simulink model "ds1_inter"  (R2019a)
settings: Solver=ode14x  StartTime=beginTime  StopTime=0.166  FixedStep=1e-4  RelTol=1e-3  EnableMultiTasking=on
model workspace (MAT data in the model file):
  Ankle_L_D = 0.125126243033
  Ankle_L_S = 0.0328154604487
  Ankle_R_D = 0.245807097642
  Ankle_R_S = 0.0328154604487
  F_C = 0.0618
  F_H = 0.107
  F_I = 0.0103200285075
  F_L = 0.2471
  F_M = 1.2499
  F_W = 0.11
  GRF_HD = 941.037069119
  GRF_HS = 1691.11560066
  GRF_VD = 12300.8672242
  GRF_VS = 76710.3574634
  HAT_I = 5.06801
  HAT_L = 0.549
  HAT_M = 58.9182
  HAT_a = 0.2
  HAT_b = 0.13
  Hip_L_D = 0.0332143791481
  Hip_L_S = 0.0516603438036
  Hip_R_D = 0.145088103411
  Hip_R_S = 0.15911410017
  Knee_L_D = 0.0558982452805
  Knee_L_S = 0.00250387295429
  Knee_R_D = 0.0619293882143
  Knee_R_S = 0.0623339259595
  M : struct (value not decoded)
  Planar_joint_x_p_i = 0
  Planar_joint_x_v_i = 0
  Planar_joint_y_p_i = 0
  Planar_joint_y_v_i = 0
  Planar_joint_z_p_i = -10.3139246991
  Planar_joint_z_w_i = -47.4942945829
  S_I = 0.0584148214017
  S_L = 0.447
  S_M = 4.0083
  S_R1 = 0.06
  S_R2 = 0.08
  T_I = 0.243990929891
  T_L = 0.476
  T_M = 8.62
  T_R1 = 0.08
  T_R2 = 0.1
  beginTime = 0
  bodymass = 86.2
  lagStanceAnkle = [0 0 0 0 0 0]
  lagStanceKnee = [0 0 0 0 0 0]
  lagSwingAnkle = [0 0 0 0 0 0]
  lagSwingKnee = [0 0 0 0 0 0]
  p_stance_ankle_i = 14.9539905036
  p_stance_hip_i = -24.9413676415
  p_stance_knee_i = -2.50807459996
  p_swing_ankle_i = 4.11757124464
  p_swing_hip_i = 18.3000604838
  p_swing_knee_i = -3.41741510381
  polyfit_stance_ankle = [-863347.977095 222377.922877 -7468.35453889 -9.40558010807 -153.06789694]
  polyfit_stance_hip = [-279786636.688 114363391.625 -15725654.0525 856134.662579 -22930.0516399 481.110496147 63.2694363354]
  polyfit_stance_knee = [-122862314.114 52903969.6705 -7988612.27678 487806.049871 -8969.32141641 330.337585729 -54.0526736443]
  polyfit_swing_ankle = [49510154320.8 -30205907167.6 7312588550.85 -888915044.437 56385922.5861 -1769074.37171 25613.4020917 -113.306543933 -1.03720591697]
  polyfit_swing_hip = [538683495113 -366532634246 101719653645 -14750073882.9 1184454520.37 -50949861.1242 1019832.60417 -6310.84925925 -38.0907282261]
  polyfit_swing_knee = [352478408737 -233011269241 62650744932.5 -8775138187.04 678489689.503 -28060179.8998 545151.783137 -3282.03325692 -26.455631467]
  time = [0 0.00833333333333 0.0166666666667 0.025 0.0333333333333 0.0416666666667 0.05 0.0583333333333 0.0666666666667 0.075 0.0833333333333 0.0916666666667 ... (21 elements, 21x1)]
  w_stance_ankle_i = 4.51440934049
  w_stance_hip_i = 2.37738035886
  w_stance_knee_i = 12.74290384
  w_swing_ankle_i = -56.5478745686
  w_swing_hip_i = 68.5572835202
  w_swing_knee_i = 17.3722348151
values from neighbouring files (symbols this model uses):
  N = 3    [lagdmodel.m]
symbols that are objects in the model workspace (value not decoded): M
undefined symbols (not defined in the file or in its folder): X, Y, Z
libraries: nesl_utility x59, sm_lib x49, fl_lib x24, fl_ps_legacy_lib x14, simulink x4
(part 2 of 3)

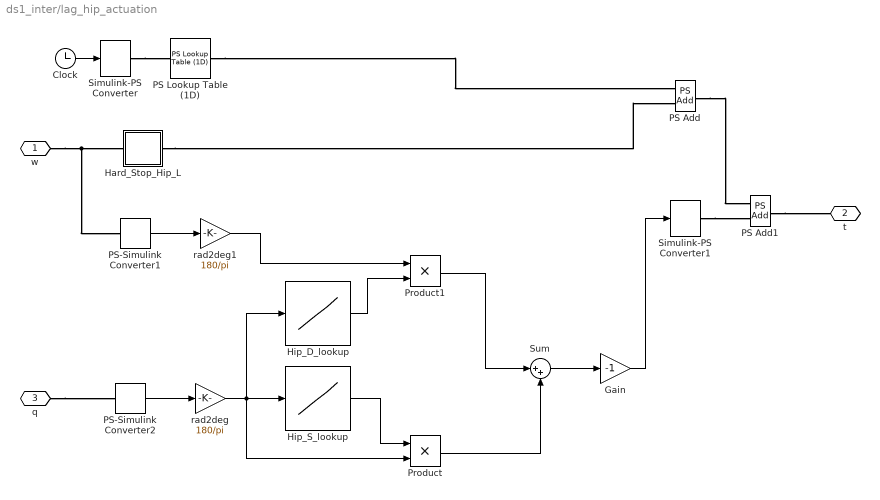
== system ds1_inter/lag_hip_actuation ==
  Clock : Clock
  Gain : Gain  Gain=-1
  Hard_Stop_Hip_L : Subsystem  mask{upper_bound=((125-p_stance_hip_i)*pi)/180, lower_bound=((-30-p_stance_hip_i)*pi)/180, contact_stiffness=1e8, contact_damping=5000, initial_angular_position=0}
      mask prompts: upper_bound "Upper Bound"; lower_bound "Lower Bound"; contact_stiffness "Contact Stiffness"; contact_damping "Contact Damping"; initial_angular_position "Initial Angular Position"
  Hip_D_lookup : Lookup_n-D  NumberOfTableDimensions=1  BreakpointsForDimension1=[-30:.01:125]  Table=[exp(linspace(log(1000),log(.01),1000)), zeros(1,13500),exp(linspace(log(.01),log(1000),1001))]  RndMeth=Simplest  InputSameDT=on
  Hip_S_lookup : Lookup_n-D  NumberOfTableDimensions=1  BreakpointsForDimension1=[-30:.01:125]  Table=[exp(linspace(log(10000),log(.01),1000)), zeros(1,13500),exp(linspace(log(.01),log(10000),1001))]  RndMeth=Simplest  InputSameDT=on
  PS Add : fl_ps_legacy_lib/Legacy Physical Signals/Functions/PS Add
      settings: SourceProductName=Simscape  SourceProductBaseCode=SS
  PS Add1 : fl_ps_legacy_lib/Legacy Physical Signals/Functions/PS Add
      settings: SourceProductName=Simscape  SourceProductBaseCode=SS
  PS Lookup Table (1D) : fl_ps_legacy_lib/Legacy Physical Signals/Lookup Tables/PS Lookup Table (1D)  x=linspace(0,.1667,21)'  f=(-M.stance_hip/1000)*bodymass  interp_method=2  extrap_method=1
      settings: SourceProductName=Simscape  SourceProductBaseCode=SS
  PS-Simulink Converter1 : nesl_utility/PS-Simulink Converter  PhysicalDomain=network_engine_domain  SubClassName=ps_output  LeftPortType=input  RightPortType=output  PseudoPeriodic=off  Frequencies=[]  Unit=1  AffineConversion=off
  PS-Simulink Converter2 : nesl_utility/PS-Simulink Converter  PhysicalDomain=network_engine_domain  SubClassName=ps_output  LeftPortType=input  RightPortType=output  PseudoPeriodic=off  Frequencies=[]  Unit=1  AffineConversion=off
  Product : Product  RndMeth=Zero
  Product1 : Product  RndMeth=Zero
  Simulink-PS Converter : nesl_utility/Simulink-PS Converter  PhysicalDomain=network_engine_domain  SubClassName=ps_input  LeftPortType=input  RightPortType=output  PseudoPeriodic=off  Frequencies=[]  NoiseDistribution=none  NoiseParameters=[]  Unit=1  AffineConversion=off  FilteringAndDerivatives=zero  SimscapeFilterOrder=1  InputFilterTimeConstant=.001  UdotUserProvided=[]
  Simulink-PS Converter1 : nesl_utility/Simulink-PS Converter  PhysicalDomain=network_engine_domain  SubClassName=ps_input  LeftPortType=input  RightPortType=output  PseudoPeriodic=off  Frequencies=[]  NoiseDistribution=none  NoiseParameters=[]  Unit=1  AffineConversion=off  FilteringAndDerivatives=zero  SimscapeFilterOrder=1  InputFilterTimeConstant=.001  UdotUserProvided=[]
  Sum : Sum  Inputs=|++
  rad2deg : Gain  Gain=180/pi
  "rad2deg1 " : Gain  Gain=180/pi
  w : PMIOPort  Side=Right
  t : PMIOPort  Port=2  Side=Left
  q : PMIOPort  Port=3  Side=Right
  wires:
  PS-Simulink Converter1/1 -> "rad2deg1 "/1
  PS-Simulink Converter2/1 -> rad2deg/1
  rad2deg/1 -> Hip_S_lookup/1, Hip_D_lookup/1, Product/2
  Hip_S_lookup/1 -> Product/1
  "rad2deg1 "/1 -> Product1/1
  Product1/1 -> Sum/1
  Product/1 -> Sum/2
  Sum/1 -> Gain/1
  Gain/1 -> Simulink-PS Converter1/1
  Hip_D_lookup/1 -> Product1/2
  Clock/1 -> Simulink-PS Converter/1
  connections:
  w/RConn1 -- PS-Simulink Converter1/LConn1 -- Hard_Stop_Hip_L/LConn1
  Hard_Stop_Hip_L/RConn1 -- PS Add/LConn2
  q/RConn1 -- PS-Simulink Converter2/LConn1
  PS Add1/RConn1 -- t/RConn1
  PS Add/RConn1 -- PS Add1/LConn1
  Simulink-PS Converter1/RConn1 -- PS Add1/LConn2
  PS Lookup Table (1D)/RConn1 -- PS Add/LConn1
  Simulink-PS Converter/RConn1 -- PS Lookup Table (1D)/LConn1

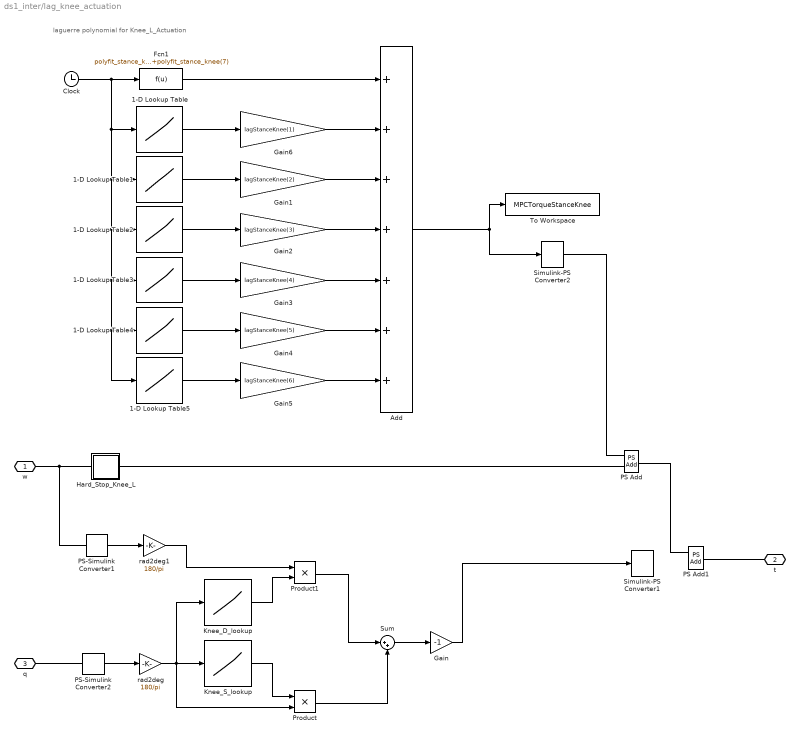
== system ds1_inter/lag_knee_actuation ==
  note: laguerre polynomial for Knee_L_Actuation
  1-D Lookup Table : Lookup_n-D  NumberOfTableDimensions=1  BreakpointsForDimension1=0:0.166/20:0.166  Table="[0.999949998749938\t0.00999949998749938\t9.99949998749938e-05\t9.99949998749938e-07\t9.99949998749938e-09\t9.99949998749938e-11\t9.99949998749938e-13\t9.99949998749938e-15\t9.99949998749938e-17\t9.99949998749938e-19\t9.99949998749938e-21\t9.99949998749938e-23\t9.99949998749938e-25\t9.99949998749938e-27\t9.99949998749938e-29\t9.99949998749938e-31\t9.99949998749938e-33\t9.99949998749938e-35\t9.99949998749938e-37\t9.99949998749938e-39\t9.99949998749938e-41]"  InternalRulePriority=Speed  RndMeth=Simplest  InputSameDT=on
  1-D Lookup Table1 : Lookup_n-D  NumberOfTableDimensions=1  BreakpointsForDimension1=0:0.166/20:0.166  Table="[-0.00999949998749938\t0.999750008750188\t0.0199960001250025\t0.000299945001625031\t3.99930002000038e-06\t4.99915002375044e-08\t5.99900002750050e-10\t6.99885003125056e-12\t7.99870003500063e-14\t8.99855003875069e-16\t9.99840004250075e-18\t1.09982500462508e-19\t1.19981000500009e-21\t1.29979500537509e-23\t1.39978000575010e-25\t1.49976500612511e-27\t1.59975000650011e-29\t1.69973500687512e-31\t1.79972000725013e-33\t1.89970500762513e-35\t1.99969000800014e-37]"  InternalRulePriority=Speed  RndMeth=Simplest  InputSameDT=on
  1-D Lookup Table2 : Lookup_n-D  NumberOfTableDimensions=1  BreakpointsForDimension1=0:0.166/20:0.166  Table="[9.99949998749938e-05\t-0.0199960001250025\t0.999350088747688\t0.0299865015624631\t0.000599770024249463\t9.99650034749263e-06\t1.49950504712403e-07\t2.09933506137377e-09\t2.79914007749848e-11\t3.59892009549815e-13\t4.49867511537279e-15\t5.49840513712241e-17\t6.59811016074699e-19\t7.79779018624654e-21\t9.09744521362106e-23\t1.04970752428705e-24\t1.19966802739950e-26\t1.35962603069944e-28\t1.52958153418688e-30\t1.70953453786182e-32\t1.89948504172425e-34]"  InternalRulePriority=Speed  RndMeth=Simplest  InputSameDT=on
  1-D Lookup Table3 : Lookup_n-D  NumberOfTableDimensions=1  BreakpointsForDimension1=0:0.166/20:0.166  Table="[-9.99949998749938e-07\t0.000299945001625031\t-0.0299865015624631\t0.998750358716438\t0.0399680074493850\t0.000999350133739838\t1.99885021798439e-05\t3.49814533160228e-07\t5.59720047896830e-09\t8.39598066445723e-11\t1.19944508924438e-12\t1.64925761673029e-14\t2.19903214934093e-16\t2.85876518751376e-18\t3.63845323168628e-20\t4.54809278229596e-22\t5.59768033978027e-24\t6.79721240457670e-26\t8.15668547712273e-28\t9.68609605785582e-30\t1.13954406472135e-31]"  InternalRulePriority=Speed  RndMeth=Simplest  InputSameDT=on
  1-D Lookup Table4 : Lookup_n-D  NumberOfTableDimensions=1  BreakpointsForDimension1=0:0.166/20:0.166  Table="[9.99949998749938e-09\t-3.99930002000038e-06\t0.000599770024249463\t-0.0399680074493850\t0.997950998567451\t0.0499375239337221\t0.00149852548805526\t3.49702589150649e-05\t6.99461150306087e-07\t1.25909723839627e-08\t2.09857536033307e-10\t3.29785552381578e-12\t4.94689323733114e-14\t7.14563951015331e-16\t1.00040408523439e-17\t1.36420392747520e-19\t1.81895722890139e-21\t2.37865729075538e-23\t3.05829696435827e-25\t3.87386865110997e-27\t4.84236430248908e-29]"  InternalRulePriority=Speed  RndMeth=Simplest  InputSameDT=on
  1-D Lookup Table5 : Lookup_n-D  NumberOfTableDimensions=1  BreakpointsForDimension1=0:0.166/20:0.166  Table="[-9.99949998749938e-11\t4.99915002375044e-08\t-9.99650034749263e-06\t0.000999350133739838\t-0.0499375239337221\t0.996952248088776\t0.0598920611597293\t0.00209709639706340\t5.59342282741959e-05\t1.25867752332421e-06\t2.51756490418445e-08\t4.61581047896514e-10\t7.91317131345719e-12\t1.28593499868373e-13\t2.00039890929054e-15\t3.00066657413218e-17\t4.36468860588449e-19\t6.18340796905681e-21\t8.56175943011575e-23\t1.16196690076089e-24\t1.54930534222886e-26]"  InternalRulePriority=Speed  RndMeth=Simplest  InputSameDT=on
  Add : Sum  Inputs=+++++++
  Clock : Clock
  Fcn1 : Fcn  Expr=polyfit_stance_knee(1)*u^6+polyfit_stance_knee(2)*u^5+polyfit_stance_knee(3)*u^4+polyfit_stance_knee(4)*u^3+polyfit_stance_knee(5)*u^2+polyfit_stance_knee(6)*u+polyfit_stance_knee(7)
  Gain : Gain  Gain=-1
  Gain1 : Gain  Gain=lagStanceKnee(2)
  Gain2 : Gain  Gain=lagStanceKnee(3)
  Gain3 : Gain  Gain=lagStanceKnee(4)
  Gain4 : Gain  Gain=lagStanceKnee(5)
  Gain5 : Gain  Gain=lagStanceKnee(6)
  Gain6 : Gain  Gain=lagStanceKnee(1)
  Hard_Stop_Knee_L : Subsystem  mask{upper_bound=(-p_stance_knee_i*pi)/180, lower_bound=((-140-p_stance_knee_i)*pi)/180, contact_stiffness=1e8, contact_damping=5000, initial_angular_position=0}
      mask prompts: upper_bound "Upper Bound"; lower_bound "Lower Bound"; contact_stiffness "Contact Stiffness"; contact_damping "Contact Damping"; initial_angular_position "Initial Angular Position"
  Knee_D_lookup : Lookup_n-D  NumberOfTableDimensions=1  BreakpointsForDimension1=[-140:.01:0]  Table=[exp(linspace(log(1000),log(.01),1000)), zeros(1,12000),exp(linspace(log(.01),log(1000),1001))]  RndMeth=Simplest  InputSameDT=on
  Knee_S_lookup : Lookup_n-D  NumberOfTableDimensions=1  BreakpointsForDimension1=[-140:.01:0]  Table=[exp(linspace(log(10000),log(.01),1000)), zeros(1,12000),exp(linspace(log(.01),log(10000),1001))]  RndMeth=Simplest  InputSameDT=on
  PS Add : fl_ps_legacy_lib/Legacy Physical Signals/Functions/PS Add
      settings: SourceProductName=Simscape  SourceProductBaseCode=SS
  PS Add1 : fl_ps_legacy_lib/Legacy Physical Signals/Functions/PS Add
      settings: SourceProductName=Simscape  SourceProductBaseCode=SS
  PS-Simulink Converter1 : nesl_utility/PS-Simulink Converter  PhysicalDomain=network_engine_domain  SubClassName=ps_output  LeftPortType=input  RightPortType=output  PseudoPeriodic=off  Frequencies=[]  Unit=1  AffineConversion=off
  PS-Simulink Converter2 : nesl_utility/PS-Simulink Converter  PhysicalDomain=network_engine_domain  SubClassName=ps_output  LeftPortType=input  RightPortType=output  PseudoPeriodic=off  Frequencies=[]  Unit=1  AffineConversion=off
  Product : Product  RndMeth=Zero
  Product1 : Product  RndMeth=Zero
  Simulink-PS Converter1 : nesl_utility/Simulink-PS Converter  PhysicalDomain=network_engine_domain  SubClassName=ps_input  LeftPortType=input  RightPortType=output  PseudoPeriodic=off  Frequencies=[]  NoiseDistribution=none  NoiseParameters=[]  Unit=1  AffineConversion=off  FilteringAndDerivatives=zero  SimscapeFilterOrder=1  InputFilterTimeConstant=.001  UdotUserProvided=[]
  Simulink-PS Converter2 : nesl_utility/Simulink-PS Converter  PhysicalDomain=network_engine_domain  SubClassName=ps_input  LeftPortType=input  RightPortType=output  PseudoPeriodic=off  Frequencies=[]  NoiseDistribution=none  NoiseParameters=[]  Unit=1  AffineConversion=off  FilteringAndDerivatives=zero  SimscapeFilterOrder=1  InputFilterTimeConstant=.001  UdotUserProvided=[]
  Sum : Sum  Inputs=|++
  To Workspace : ToWorkspace  VariableName=MPCTorqueStanceKnee  SampleTime=-1
  rad2deg : Gain  Gain=180/pi
  "rad2deg1 " : Gain  Gain=180/pi
  w : PMIOPort  Side=Right
  t : PMIOPort  Port=2  Side=Left
  q : PMIOPort  Port=3  Side=Right
  wires:
  PS-Simulink Converter1/1 -> "rad2deg1 "/1
  PS-Simulink Converter2/1 -> rad2deg/1
  rad2deg/1 -> Knee_S_lookup/1, Knee_D_lookup/1, Product/2
  Knee_S_lookup/1 -> Product/1
  "rad2deg1 "/1 -> Product1/1
  Product1/1 -> Sum/1
  Product/1 -> Sum/2
  Sum/1 -> Gain/1
  Gain/1 -> Simulink-PS Converter1/1
  Knee_D_lookup/1 -> Product1/2
  Add/1 -> To Workspace/1, Simulink-PS Converter2/1
  Gain5/1 -> Add/7
  1-D Lookup Table5/1 -> Gain5/1
  Gain4/1 -> Add/6
  1-D Lookup Table4/1 -> Gain4/1
  Gain3/1 -> Add/5
  1-D Lookup Table3/1 -> Gain3/1
  Gain2/1 -> Add/4
  1-D Lookup Table2/1 -> Gain2/1
  Gain1/1 -> Add/3
  1-D Lookup Table1/1 -> Gain1/1
  Gain6/1 -> Add/2
  1-D Lookup Table/1 -> Gain6/1
  Fcn1/1 -> Add/1
  Clock/1 -> 1-D Lookup Table2/1, 1-D Lookup Table5/1, 1-D Lookup Table4/1, 1-D Lookup Table3/1, 1-D Lookup Table1/1, 1-D Lookup Table/1, Fcn1/1
  connections:
  w/RConn1 -- PS-Simulink Converter1/LConn1 -- Hard_Stop_Knee_L/LConn1
  t/RConn1 -- PS Add1/RConn1
  q/RConn1 -- PS-Simulink Converter2/LConn1
  PS Add/RConn1 -- PS Add1/LConn1
  Hard_Stop_Knee_L/RConn1 -- PS Add/LConn2
  Simulink-PS Converter2/RConn1 -- PS Add/LConn1

== system ds1_inter/lag_planar ==
  Planar Joint : sm_lib/Joints/Planar Joint  SenseConstraintForce=off  SenseConstraintForceX=off  SenseConstraintForceY=off  SenseConstraintForceZ=off  SenseConstraintTorque=off  SenseConstraintTorqueX=off  SenseConstraintTorqueY=off  SenseConstraintTorqueZ=off  SenseTotalForce=off  SenseTotalForceX=off  SenseTotalForceY=off  SenseTotalForceZ=off  SenseTotalTorque=off  SenseTotalTorqueX=off  SenseTotalTorqueY=off  SenseTotalTorqueZ=off  CompositeWrenchDir=FollowerOnBase  CompositeWrenchFrame=BaseFrame  PxEquilibriumPosition=0  PxEquilibriumPositionUnits=m  PxSpringStiffness=0  PxSpringStiffnessUnits=N/m  PxDampingCoefficient=0  PxDampingCoefficientUnits=N/(m/s)  PxTorqueActuationMode=NoTorque  PxMotionActuationMode=ComputedMotion  PxSensePosition=off  PxSenseVelocity=off  PxSenseAcceleration=off  PxSenseTorqueForce=off  PxSenseLowerLimitTorqueForce=off  PxSenseUpperLimitTorqueForce=off  PxLowerLimitSpecify=off  PxLowerLimitBound=-1  PxLowerLimitBoundUnits=m  PxLowerLimitStiffness=1e6  PxLowerLimitStiffnessUnits=N/m  PxLowerLimitDamping=1e3  PxLowerLimitDampingUnits=N/(m/s)  PxLowerLimitTransitionRegionWidth=1e-4  PxLowerLimitTransitionRegionWidthUnits=m  PxUpperLimitSpecify=off  PxUpperLimitBound=1  PxUpperLimitBoundUnits=m  PxUpperLimitStiffness=1e6  PxUpperLimitStiffnessUnits=N/m  PxUpperLimitDamping=1e3  PxUpperLimitDampingUnits=N/(m/s)  PxUpperLimitTransitionRegionWidth=1e-4  PxUpperLimitTransitionRegionWidthUnits=m  PxPositionTargetSpecify=on  PxPositionTargetPriority=High  PxPositionTargetValue=Planar_joint_x_p_i  PxPositionTargetValueUnits=m  PxVelocityTargetSpecify=on  PxVelocityTargetPriority=High  PxVelocityTargetValue=Planar_joint_x_v_i  PxVelocityTargetValueUnits=m/s  PyEquilibriumPosition=0  PyEquilibriumPositionUnits=m  PySpringStiffness=0  PySpringStiffnessUnits=N/m  PyDampingCoefficient=0  PyDampingCoefficientUnits=N/(m/s)  PyTorqueActuationMode=NoTorque  PyMotionActuationMode=ComputedMotion  PySensePosition=off  PySenseVelocity=off  PySenseAcceleration=off  PySenseTorqueForce=off  PySenseLowerLimitTorqueForce=off  PySenseUpperLimitTorqueForce=off  PyLowerLimitSpecify=off  PyLowerLimitBound=-1  PyLowerLimitBoundUnits=m  PyLowerLimitStiffness=1e6  PyLowerLimitStiffnessUnits=N/m  PyLowerLimitDamping=1e3  PyLowerLimitDampingUnits=N/(m/s)  PyLowerLimitTransitionRegionWidth=1e-4  PyLowerLimitTransitionRegionWidthUnits=m  PyUpperLimitSpecify=off  PyUpperLimitBound=1  PyUpperLimitBoundUnits=m  PyUpperLimitStiffness=1e6  PyUpperLimitStiffnessUnits=N/m  PyUpperLimitDamping=1e3  PyUpperLimitDampingUnits=N/(m/s)  PyUpperLimitTransitionRegionWidth=1e-4  PyUpperLimitTransitionRegionWidthUnits=m  PyPositionTargetSpecify=on  PyPositionTargetPriority=High  PyPositionTargetValue=Planar_joint_y_p_i  PyPositionTargetValueUnits=m  PyVelocityTargetSpecify=on  PyVelocityTargetPriority=High  PyVelocityTargetValue=Planar_joint_y_v_i  PyVelocityTargetValueUnits=m/s  RzEquilibriumPosition=0  RzEquilibriumPositionUnits=deg  RzSpringStiffness=0  RzSpringStiffnessUnits=N*m/deg  RzDampingCoefficient=0  RzDampingCoefficientUnits=N*m/(deg/s)  RzTorqueActuationMode=NoTorque  RzMotionActuationMode=ComputedMotion  RzSensePosition=off  RzSenseVelocity=off  RzSenseAcceleration=off  RzSenseTorqueForce=off  RzSenseLowerLimitTorqueForce=off  RzSenseUpperLimitTorqueForce=off  RzLowerLimitSpecify=off  RzLowerLimitBound=-90  RzLowerLimitBoundUnits=deg  RzLowerLimitStiffness=1e4  RzLowerLimitStiffnessUnits=N*m/deg  RzLowerLimitDamping=10  RzLowerLimitDampingUnits=N*m/(deg/s)  RzLowerLimitTransitionRegionWidth=0.1  RzLowerLimitTransitionRegionWidthUnits=deg  RzUpperLimitSpecify=off  RzUpperLimitBound=90  RzUpperLimitBoundUnits=deg  RzUpperLimitStiffness=1e4  RzUpperLimitStiffnessUnits=N*m/deg  RzUpperLimitDamping=10  RzUpperLimitDampingUnits=N*m/(deg/s)  RzUpperLimitTransitionRegionWidth=0.1  RzUpperLimitTransitionRegionWidthUnits=deg  RzPositionTargetSpecify=on  RzPositionTargetPriority=High  RzPositionTargetValue=Planar_joint_z_p_i  RzPositionTargetValueUnits=deg  RzVelocityTargetSpecify=on  RzVelocityTargetPriority=High  RzVelocityTargetValue=Planar_joint_z_w_i  RzVelocityTargetValueUnits=deg/s
  Rigid  Transform : sm_lib/Frames and Transforms/Rigid Transform  TranslationMethod=StandardAxis  TranslationStandardOffset=F_L-F_C  TranslationLengthUnit=m  TranslationStandardAxis=+Y  TranslationCartesianOffset=[0 0 0]  TranslationROffset=0  TranslationROffsetUnits=m  TranslationZOffset=0  TranslationZOffsetUnits=m  TranslationThetaOffset=0  TranslationThetaOffsetUnits=deg  RotationMethod=AlignedAxes  RotationAngleUnits=deg  RotationStandardAxis=+Z  RotationAngle=0  RotationArbitraryAxis=[0 0 1]  FollAlignAxisA=+X  BaseAlignAxisA=+Y  FollAlignAxisB=+Y  BaseAlignAxisB=+Z  RotationSequenceAxes=FollowerAxes  RotationSequence=XYX  RotationSequenceAngles=[0 0 0]  RotationSequenceAnglesUnits=deg  RotationMatrix=[1 0 0; 0 1 0; 0 0 1]
  Rigid  Transform1 : sm_lib/Frames and Transforms/Rigid Transform  TranslationMethod=StandardAxis  TranslationStandardOffset=F_L-F_C  TranslationLengthUnit=m  TranslationStandardAxis=-X  TranslationCartesianOffset=[0 0 0]  TranslationROffset=0  TranslationROffsetUnits=m  TranslationZOffset=0  TranslationZOffsetUnits=m  TranslationThetaOffset=0  TranslationThetaOffsetUnits=deg  RotationMethod=AlignedAxes  RotationAngleUnits=deg  RotationStandardAxis=+Z  RotationAngle=0  RotationArbitraryAxis=[0 0 1]  FollAlignAxisA=+Z  BaseAlignAxisA=+Y  FollAlignAxisB=+X  BaseAlignAxisB=+Z  RotationSequenceAxes=FollowerAxes  RotationSequence=XYX  RotationSequenceAngles=[0 0 0]  RotationSequenceAnglesUnits=deg  RotationMatrix=[1 0 0; 0 1 0; 0 0 1]
  B : PMIOPort  Side=Left
  F : PMIOPort  Port=2  Side=Right
  connections:
  Rigid  Transform1/RConn1 -- F/RConn1
  Rigid  Transform/LConn1 -- B/RConn1
  Rigid  Transform/RConn1 -- Planar Joint/LConn1
  Planar Joint/RConn1 -- Rigid  Transform1/LConn1

== system ds1_inter/lead foot ==
  Ankle_L : sm_lib/Frames and Transforms/Rigid Transform  TranslationMethod=StandardAxis  TranslationStandardOffset=F_H  TranslationLengthUnit=m  TranslationStandardAxis=+Y  TranslationCartesianOffset=[0 0 0]  TranslationROffset=0  TranslationROffsetUnits=m  TranslationZOffset=0  TranslationZOffsetUnits=m  TranslationThetaOffset=0  TranslationThetaOffsetUnits=deg  RotationMethod=StandardAxis  RotationAngleUnits=deg  RotationStandardAxis=+Z  RotationAngle=-90  RotationArbitraryAxis=[0 0 1]  FollAlignAxisA=+Z  BaseAlignAxisA=+Z  FollAlignAxisB=+X  BaseAlignAxisB=+Y  RotationSequenceAxes=FollowerAxes  RotationSequence=XYX  RotationSequenceAngles=[0 0 0]  RotationSequenceAnglesUnits=deg  RotationMatrix=[1 0 0; 0 1 0; 0 0 1]
  Heel : sm_lib/Frames and Transforms/Rigid Transform  TranslationMethod=StandardAxis  TranslationStandardOffset=F_C  TranslationLengthUnit=m  TranslationStandardAxis=-X  TranslationCartesianOffset=[0 0 0]  TranslationROffset=0  TranslationROffsetUnits=m  TranslationZOffset=0  TranslationZOffsetUnits=m  TranslationThetaOffset=0  TranslationThetaOffsetUnits=deg  RotationMethod=AlignedAxes  RotationAngleUnits=deg  RotationStandardAxis=+Z  RotationAngle=0  RotationArbitraryAxis=[0 0 1]  FollAlignAxisA=+X  BaseAlignAxisA=+Z  FollAlignAxisB=+Y  BaseAlignAxisB=+X  RotationSequenceAxes=FollowerAxes  RotationSequence=XYX  RotationSequenceAngles=[0 0 0]  RotationSequenceAnglesUnits=deg  RotationMatrix=[1 0 0; 0 1 0; 0 0 1]
  Heel_GRF : Subsystem
  Rigid  Transform : sm_lib/Frames and Transforms/Rigid Transform  TranslationMethod=StandardAxis  TranslationStandardOffset=T_R2  TranslationLengthUnit=m  TranslationStandardAxis=+Z  TranslationCartesianOffset=[0 0 0]  TranslationROffset=0  TranslationROffsetUnits=m  TranslationZOffset=0  TranslationZOffsetUnits=m  TranslationThetaOffset=0  TranslationThetaOffsetUnits=deg  RotationMethod=AlignedAxes  RotationAngleUnits=deg  RotationStandardAxis=+Z  RotationAngle=0  RotationArbitraryAxis=[0 0 1]  FollAlignAxisA=+X  BaseAlignAxisA=+Z  FollAlignAxisB=+Z  BaseAlignAxisB=+Y  RotationSequenceAxes=FollowerAxes  RotationSequence=XYX  RotationSequenceAngles=[0 0 0]  RotationSequenceAnglesUnits=deg  RotationMatrix=[1 0 0; 0 1 0; 0 0 1]
  Solid : sm_lib/Body Elements/Solid  InertiaType=Custom  Mass=F_M  MassUnits=kg  CenterOfMass=[(F_L-F_C)/2, F_H/2, 0]  CenterOfMassUnits=m  MomentsOfInertia=[0.001 0.001 F_I]  MomentsOfInertiaUnits=kg*m^2  ProductsOfInertia=[0 0 0]  ProductsOfInertiaUnits=kg*m^2  BasedOnType=Density  Density=0  DensityUnits=kg/(m^3)  DoExposeReferenceFrame=on  SerializedFrames=<Frames/>  GraphicType=FromGeometry  MarkerShape=Sphere  MarkerSize=10  MarkerSizeUnits=m  GraphicVisPropType=SimpleVisualProperties  GraphicDiffuseColor=[0.0 0.4 1.0]  GraphicSpecularColor=[0.5 0.5 0.5 1.0]  GraphicAmbientColor=[0.15 0.15 0.15 1.0]  GraphicEmissiveColor=[0.0 0.0 0.0 1.0]  GraphicShininess=75  GraphicOpacity=1.0  GeometryShape=GeneralExtrusion  RectangleSize=[1 1]  RectangleSizeUnits=m  BrickDimensions=[1 1 1]  BrickDimensionUnits=m  CylinderRadius=1  CylinderRadiusUnits=m  CylinderLength=1  CylinderLengthUnits=m  SphereRadius=1  SphereRadiusUnits=m  EllipsoidRadii=[1 1 1]  EllipsoidRadiiUnits=m  ExtrusionCrossSection=F_cross_section  ExtrusionCrossSectionUnits=m  ExtrusionLength=F_W  ExtrusionLengthUnits=m  PolygonNumSides=3  PolygonOuterRadius=1  PolygonOuterRadiusUnits=m  ExtGeomFileType=STEP  ExtGeomFileUnits=m  RevolutionCrossSection=[1 1; 1 -1; 2 -1; 2 1]  RevolutionCrossSectionUnits=m  RevolutionExtent=Full  RevolutionAngle=180  RevolutionAngleUnits=deg
  Toe : sm_lib/Frames and Transforms/Rigid Transform  TranslationMethod=StandardAxis  TranslationStandardOffset=F_L-F_C  TranslationLengthUnit=m  TranslationStandardAxis=+X  TranslationCartesianOffset=[0 0 0]  TranslationROffset=0  TranslationROffsetUnits=m  TranslationZOffset=0  TranslationZOffsetUnits=m  TranslationThetaOffset=0  TranslationThetaOffsetUnits=deg  RotationMethod=AlignedAxes  RotationAngleUnits=deg  RotationStandardAxis=+Z  RotationAngle=0  RotationArbitraryAxis=[0 0 1]  FollAlignAxisA=+X  BaseAlignAxisA=+Z  FollAlignAxisB=+Y  BaseAlignAxisB=+X  RotationSequenceAxes=FollowerAxes  RotationSequence=XYX  RotationSequenceAngles=[0 0 0]  RotationSequenceAnglesUnits=deg  RotationMatrix=[1 0 0; 0 1 0; 0 0 1]
  "Toe_GRF " : Subsystem
  B : PMIOPort  Side=Right
  F : PMIOPort  Port=2  Side=Left
  connections:
  B/RConn1 -- Rigid  Transform/RConn1
  Rigid  Transform/LConn1 -- Ankle_L/LConn1 -- Toe/LConn1 -- Heel/LConn1 -- Solid/RConn1
  Ankle_L/RConn1 -- F/RConn1
  Heel/RConn1 -- Heel_GRF/LConn1
  Toe/RConn1 -- "Toe_GRF "/LConn1

== system ds1_inter/lead shank ==
  Rigid  Transform : sm_lib/Frames and Transforms/Rigid Transform  TranslationMethod=None  TranslationStandardOffset=S_L  TranslationLengthUnit=m  TranslationStandardAxis=+Z  TranslationCartesianOffset=[0 0 0]  TranslationROffset=0  TranslationROffsetUnits=m  TranslationZOffset=0  TranslationZOffsetUnits=m  TranslationThetaOffset=0  TranslationThetaOffsetUnits=deg  RotationMethod=StandardAxis  RotationAngleUnits=deg  RotationStandardAxis=+Y  RotationAngle=90  RotationArbitraryAxis=[0 0 1]  FollAlignAxisA=+X  BaseAlignAxisA=+Y  FollAlignAxisB=+Y  BaseAlignAxisB=+Z  RotationSequenceAxes=FollowerAxes  RotationSequence=XYX  RotationSequenceAngles=[0 0 0]  RotationSequenceAnglesUnits=deg  RotationMatrix=[1 0 0; 0 1 0; 0 0 1]
  Rigid  Transform1 : sm_lib/Frames and Transforms/Rigid Transform  TranslationMethod=StandardAxis  TranslationStandardOffset=S_L  TranslationLengthUnit=m  TranslationStandardAxis=+Z  TranslationCartesianOffset=[0 0 0]  TranslationROffset=0  TranslationROffsetUnits=m  TranslationZOffset=0  TranslationZOffsetUnits=m  TranslationThetaOffset=0  TranslationThetaOffsetUnits=deg  RotationMethod=StandardAxis  RotationAngleUnits=deg  RotationStandardAxis=+Y  RotationAngle=90  RotationArbitraryAxis=[0 0 1]  FollAlignAxisA=+X  BaseAlignAxisA=+Y  FollAlignAxisB=+Y  BaseAlignAxisB=+Z  RotationSequenceAxes=FollowerAxes  RotationSequence=XYX  RotationSequenceAngles=[0 0 0]  RotationSequenceAnglesUnits=deg  RotationMatrix=[1 0 0; 0 1 0; 0 0 1]
  Solid : sm_lib/Body Elements/Solid  InertiaType=Custom  Mass=S_M  MassUnits=kg  CenterOfMass=[0 0 0.567*S_L]  CenterOfMassUnits=m  MomentsOfInertia=[S_I .001 .001]  MomentsOfInertiaUnits=kg*m^2  ProductsOfInertia=[0 0 0]  ProductsOfInertiaUnits=kg*m^2  BasedOnType=Density  Density=0  DensityUnits=kg/(m^3)  DoExposeReferenceFrame=on  SerializedFrames=<Frames/>  GraphicType=FromGeometry  MarkerShape=Sphere  MarkerSize=10  MarkerSizeUnits=m  GraphicVisPropType=SimpleVisualProperties  GraphicDiffuseColor=[0.0 0.4 1.0]  GraphicSpecularColor=[0.5 0.5 0.5 1.0]  GraphicAmbientColor=[0.15 0.15 0.15 1.0]  GraphicEmissiveColor=[0.0 0.0 0.0 1.0]  GraphicShininess=75  GraphicOpacity=1.0  GeometryShape=GeneralSolidOfRevolution  RectangleSize=[1 1]  RectangleSizeUnits=m  BrickDimensions=[1 1 1]  BrickDimensionUnits=m  CylinderRadius=1  CylinderRadiusUnits=m  CylinderLength=1  CylinderLengthUnits=m  SphereRadius=1  SphereRadiusUnits=m  EllipsoidRadii=[1 1 1]  EllipsoidRadiiUnits=m  ExtrusionCrossSection=[1 1; -1 1; -1 -1; 1 -1]  ExtrusionCrossSectionUnits=m  ExtrusionLength=1  ExtrusionLengthUnits=m  PolygonNumSides=3  PolygonOuterRadius=1  PolygonOuterRadiusUnits=m  ExtGeomFileType=STEP  ExtGeomFileUnits=m  RevolutionCrossSection=S_cross_section  RevolutionCrossSectionUnits=m  RevolutionExtent=Full  RevolutionAngle=180  RevolutionAngleUnits=deg
  B : PMIOPort  Side=Right
  F : PMIOPort  Port=2  Side=Left
  connections:
  B/RConn1 -- Rigid  Transform/RConn1
  Rigid  Transform/LConn1 -- Rigid  Transform1/LConn1 -- Solid/RConn1
  F/RConn1 -- Rigid  Transform1/RConn1

== system ds1_inter/lead thigh ==
  Rigid  Transform : sm_lib/Frames and Transforms/Rigid Transform  TranslationMethod=None  TranslationStandardOffset=T_L  TranslationLengthUnit=m  TranslationStandardAxis=+Z  TranslationCartesianOffset=[0 0 0]  TranslationROffset=0  TranslationROffsetUnits=m  TranslationZOffset=0  TranslationZOffsetUnits=m  TranslationThetaOffset=0  TranslationThetaOffsetUnits=deg  RotationMethod=StandardAxis  RotationAngleUnits=deg  RotationStandardAxis=+Y  RotationAngle=90  RotationArbitraryAxis=[0 0 1]  FollAlignAxisA=+X  BaseAlignAxisA=+Y  FollAlignAxisB=+Y  BaseAlignAxisB=+Z  RotationSequenceAxes=FollowerAxes  RotationSequence=XYX  RotationSequenceAngles=[0 0 0]  RotationSequenceAnglesUnits=deg  RotationMatrix=[1 0 0; 0 1 0; 0 0 1]
  Rigid  Transform1 : sm_lib/Frames and Transforms/Rigid Transform  TranslationMethod=StandardAxis  TranslationStandardOffset=T_L  TranslationLengthUnit=m  TranslationStandardAxis=+Z  TranslationCartesianOffset=[0 0 0]  TranslationROffset=0  TranslationROffsetUnits=m  TranslationZOffset=0  TranslationZOffsetUnits=m  TranslationThetaOffset=0  TranslationThetaOffsetUnits=deg  RotationMethod=StandardAxis  RotationAngleUnits=deg  RotationStandardAxis=+Y  RotationAngle=90  RotationArbitraryAxis=[0 0 1]  FollAlignAxisA=+X  BaseAlignAxisA=+Y  FollAlignAxisB=+Y  BaseAlignAxisB=+Z  RotationSequenceAxes=FollowerAxes  RotationSequence=XYX  RotationSequenceAngles=[0 0 0]  RotationSequenceAnglesUnits=deg  RotationMatrix=[1 0 0; 0 1 0; 0 0 1]
  Thigh : sm_lib/Body Elements/Solid  InertiaType=Custom  Mass=T_M  MassUnits=kg  CenterOfMass=[0 0 0.567*T_L]  CenterOfMassUnits=m  MomentsOfInertia=[T_I .001 .001]  MomentsOfInertiaUnits=kg*m^2  ProductsOfInertia=[0 0 0]  ProductsOfInertiaUnits=kg*m^2  BasedOnType=Density  Density=0  DensityUnits=kg/(m^3)  DoExposeReferenceFrame=on  SerializedFrames=<Frames/>  GraphicType=FromGeometry  MarkerShape=Sphere  MarkerSize=10  MarkerSizeUnits=m  GraphicVisPropType=SimpleVisualProperties  GraphicDiffuseColor=[0.0 0.4 1.0]  GraphicSpecularColor=[0.5 0.5 0.5 1.0]  GraphicAmbientColor=[0.15 0.15 0.15 1.0]  GraphicEmissiveColor=[0.0 0.0 0.0 1.0]  GraphicShininess=75  GraphicOpacity=1.0  GeometryShape=GeneralSolidOfRevolution  RectangleSize=[1 1]  RectangleSizeUnits=m  BrickDimensions=[1 1 1]  BrickDimensionUnits=m  CylinderRadius=[1 2]  CylinderRadiusUnits=m  CylinderLength=1  CylinderLengthUnits=m  SphereRadius=1  SphereRadiusUnits=m  EllipsoidRadii=[1 1 1]  EllipsoidRadiiUnits=m  ExtrusionCrossSection=T_cross_section  ExtrusionCrossSectionUnits=cm  ExtrusionLength=T_L  ExtrusionLengthUnits=cm  PolygonNumSides=3  PolygonOuterRadius=1  PolygonOuterRadiusUnits=m  ExtGeomFileType=STEP  ExtGeomFileUnits=m  RevolutionCrossSection=T_cross_section  RevolutionCrossSectionUnits=m  RevolutionExtent=Full  RevolutionAngle=180  RevolutionAngleUnits=deg
  B : PMIOPort  Side=Right
  F : PMIOPort  Port=2  Side=Left
  connections:
  B/RConn1 -- Rigid  Transform/RConn1
  Rigid  Transform/LConn1 -- Rigid  Transform1/LConn1 -- Thigh/RConn1
  Rigid  Transform1/RConn1 -- F/RConn1

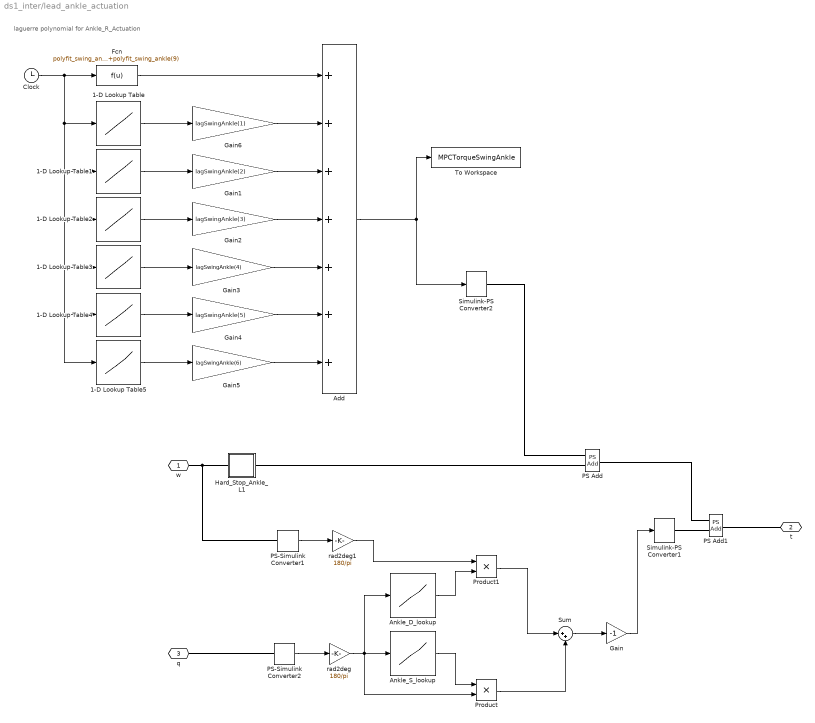
== system ds1_inter/lead_ankle_actuation ==
  note: laguerre polynomial for Ankle_R_Actuation
  1-D Lookup Table : Lookup_n-D  NumberOfTableDimensions=1  BreakpointsForDimension1=0:0.166/20:0.166  Table="[0.999949998749938\t0.00999949998749938\t9.99949998749938e-05\t9.99949998749938e-07\t9.99949998749938e-09\t9.99949998749938e-11\t9.99949998749938e-13\t9.99949998749938e-15\t9.99949998749938e-17\t9.99949998749938e-19\t9.99949998749938e-21\t9.99949998749938e-23\t9.99949998749938e-25\t9.99949998749938e-27\t9.99949998749938e-29\t9.99949998749938e-31\t9.99949998749938e-33\t9.99949998749938e-35\t9.99949998749938e-37\t9.99949998749938e-39\t9.99949998749938e-41]"  InternalRulePriority=Speed  RndMeth=Simplest  InputSameDT=on
  1-D Lookup Table1 : Lookup_n-D  NumberOfTableDimensions=1  BreakpointsForDimension1=0:0.166/20:0.166  Table="[-0.00999949998749938\t0.999750008750188\t0.0199960001250025\t0.000299945001625031\t3.99930002000038e-06\t4.99915002375044e-08\t5.99900002750050e-10\t6.99885003125056e-12\t7.99870003500063e-14\t8.99855003875069e-16\t9.99840004250075e-18\t1.09982500462508e-19\t1.19981000500009e-21\t1.29979500537509e-23\t1.39978000575010e-25\t1.49976500612511e-27\t1.59975000650011e-29\t1.69973500687512e-31\t1.79972000725013e-33\t1.89970500762513e-35\t1.99969000800014e-37]"  InternalRulePriority=Speed  RndMeth=Simplest  InputSameDT=on
  1-D Lookup Table2 : Lookup_n-D  NumberOfTableDimensions=1  BreakpointsForDimension1=0:0.166/20:0.166  Table="[9.99949998749938e-05\t-0.0199960001250025\t0.999350088747688\t0.0299865015624631\t0.000599770024249463\t9.99650034749263e-06\t1.49950504712403e-07\t2.09933506137377e-09\t2.79914007749848e-11\t3.59892009549815e-13\t4.49867511537279e-15\t5.49840513712241e-17\t6.59811016074699e-19\t7.79779018624654e-21\t9.09744521362106e-23\t1.04970752428705e-24\t1.19966802739950e-26\t1.35962603069944e-28\t1.52958153418688e-30\t1.70953453786182e-32\t1.89948504172425e-34]"  InternalRulePriority=Speed  RndMeth=Simplest  InputSameDT=on
  1-D Lookup Table3 : Lookup_n-D  NumberOfTableDimensions=1  BreakpointsForDimension1=0:0.166/20:0.166  Table="[-9.99949998749938e-07\t0.000299945001625031\t-0.0299865015624631\t0.998750358716438\t0.0399680074493850\t0.000999350133739838\t1.99885021798439e-05\t3.49814533160228e-07\t5.59720047896830e-09\t8.39598066445723e-11\t1.19944508924438e-12\t1.64925761673029e-14\t2.19903214934093e-16\t2.85876518751376e-18\t3.63845323168628e-20\t4.54809278229596e-22\t5.59768033978027e-24\t6.79721240457670e-26\t8.15668547712273e-28\t9.68609605785582e-30\t1.13954406472135e-31]"  InternalRulePriority=Speed  RndMeth=Simplest  InputSameDT=on
  1-D Lookup Table4 : Lookup_n-D  NumberOfTableDimensions=1  BreakpointsForDimension1=0:0.166/20:0.166  Table="[9.99949998749938e-09\t-3.99930002000038e-06\t0.000599770024249463\t-0.0399680074493850\t0.997950998567451\t0.0499375239337221\t0.00149852548805526\t3.49702589150649e-05\t6.99461150306087e-07\t1.25909723839627e-08\t2.09857536033307e-10\t3.29785552381578e-12\t4.94689323733114e-14\t7.14563951015331e-16\t1.00040408523439e-17\t1.36420392747520e-19\t1.81895722890139e-21\t2.37865729075538e-23\t3.05829696435827e-25\t3.87386865110997e-27\t4.84236430248908e-29]"  InternalRulePriority=Speed  RndMeth=Simplest  InputSameDT=on
  1-D Lookup Table5 : Lookup_n-D  NumberOfTableDimensions=1  BreakpointsForDimension1=0:0.166/20:0.166  Table="[-9.99949998749938e-11\t4.99915002375044e-08\t-9.99650034749263e-06\t0.000999350133739838\t-0.0499375239337221\t0.996952248088776\t0.0598920611597293\t0.00209709639706340\t5.59342282741959e-05\t1.25867752332421e-06\t2.51756490418445e-08\t4.61581047896514e-10\t7.91317131345719e-12\t1.28593499868373e-13\t2.00039890929054e-15\t3.00066657413218e-17\t4.36468860588449e-19\t6.18340796905681e-21\t8.56175943011575e-23\t1.16196690076089e-24\t1.54930534222886e-26]"  InternalRulePriority=Speed  RndMeth=Simplest  InputSameDT=on
  Add : Sum  Inputs=+++++++
  Ankle_D_lookup : Lookup_n-D  NumberOfTableDimensions=1  BreakpointsForDimension1=[-45:.01:20]  Table=[exp(linspace(log(1000),log(.01),1000)), zeros(1,4500),exp(linspace(log(.01),log(1000),1001))]  RndMeth=Simplest  InputSameDT=on
  Ankle_S_lookup : Lookup_n-D  NumberOfTableDimensions=1  BreakpointsForDimension1=[-45:.01:20]  Table=[exp(linspace(log(10000),log(.01),1000)), zeros(1,4500),exp(linspace(log(.01),log(10000),1001))]  RndMeth=Simplest  InputSameDT=on
  Clock : Clock
  Fcn : Fcn  Expr=polyfit_swing_ankle(1)*u^8+polyfit_swing_ankle(2)*u^7+polyfit_swing_ankle(3)*u^6+polyfit_swing_ankle(4)*u^5+polyfit_swing_ankle(5)*u^4+polyfit_swing_ankle(6)*u^3+polyfit_swing_ankle(7)*u^2+polyfit_swing_ankle(8)*u+polyfit_swing_ankle(9)
  Gain : Gain  Gain=-1
  Gain1 : Gain  Gain=lagSwingAnkle(2)
  Gain2 : Gain  Gain=lagSwingAnkle(3)
  Gain3 : Gain  Gain=lagSwingAnkle(4)
  Gain4 : Gain  Gain=lagSwingAnkle(5)
  Gain5 : Gain  Gain=lagSwingAnkle(6)
  Gain6 : Gain  Gain=lagSwingAnkle(1)
  Hard_Stop_Ankle_L1 : Subsystem  mask{upper_bound=((20-p_swing_ankle_i)*pi)/180, lower_bound=((-45-p_swing_ankle_i)*pi)/180, contact_stiffness=1e8, contact_damping=5000, initial_angular_position=0}
      mask prompts: upper_bound "Upper Bound"; lower_bound "Lower Bound"; contact_stiffness "Contact Stiffness"; contact_damping "Contact Damping"; initial_angular_position "Initial Angular Position"
  PS Add : fl_ps_legacy_lib/Legacy Physical Signals/Functions/PS Add
      settings: SourceProductName=Simscape  SourceProductBaseCode=SS
  PS Add1 : fl_ps_legacy_lib/Legacy Physical Signals/Functions/PS Add
      settings: SourceProductName=Simscape  SourceProductBaseCode=SS
  PS-Simulink Converter1 : nesl_utility/PS-Simulink Converter  PhysicalDomain=network_engine_domain  SubClassName=ps_output  LeftPortType=input  RightPortType=output  PseudoPeriodic=off  Frequencies=[]  Unit=1  AffineConversion=off
  PS-Simulink Converter2 : nesl_utility/PS-Simulink Converter  PhysicalDomain=network_engine_domain  SubClassName=ps_output  LeftPortType=input  RightPortType=output  PseudoPeriodic=off  Frequencies=[]  Unit=1  AffineConversion=off
  Product : Product  RndMeth=Zero
  Product1 : Product  RndMeth=Zero
  Simulink-PS Converter1 : nesl_utility/Simulink-PS Converter  PhysicalDomain=network_engine_domain  SubClassName=ps_input  LeftPortType=input  RightPortType=output  PseudoPeriodic=off  Frequencies=[]  NoiseDistribution=none  NoiseParameters=[]  Unit=1  AffineConversion=off  FilteringAndDerivatives=zero  SimscapeFilterOrder=1  InputFilterTimeConstant=.001  UdotUserProvided=[]
  Simulink-PS Converter2 : nesl_utility/Simulink-PS Converter  PhysicalDomain=network_engine_domain  SubClassName=ps_input  LeftPortType=input  RightPortType=output  PseudoPeriodic=off  Frequencies=[]  NoiseDistribution=none  NoiseParameters=[]  Unit=1  AffineConversion=off  FilteringAndDerivatives=zero  SimscapeFilterOrder=1  InputFilterTimeConstant=.001  UdotUserProvided=[]
  Sum : Sum  Inputs=|++
  To Workspace : ToWorkspace  VariableName=MPCTorqueSwingAnkle  SampleTime=-1
  rad2deg : Gain  Gain=180/pi
  "rad2deg1 " : Gain  Gain=180/pi
  w : PMIOPort  Side=Right
  t : PMIOPort  Port=2  Side=Left
  q : PMIOPort  Port=3  Side=Right
  wires:
  PS-Simulink Converter1/1 -> "rad2deg1 "/1
  PS-Simulink Converter2/1 -> rad2deg/1
  rad2deg/1 -> Ankle_D_lookup/1, Product/2, Ankle_S_lookup/1
  Ankle_S_lookup/1 -> Product/1
  "rad2deg1 "/1 -> Product1/1
  Product1/1 -> Sum/1
  Product/1 -> Sum/2
  Sum/1 -> Gain/1
  Gain/1 -> Simulink-PS Converter1/1
  Ankle_D_lookup/1 -> Product1/2
  Add/1 -> To Workspace/1, Simulink-PS Converter2/1
  Gain5/1 -> Add/7
  1-D Lookup Table5/1 -> Gain5/1
  Gain4/1 -> Add/6
  1-D Lookup Table4/1 -> Gain4/1
  Gain3/1 -> Add/5
  1-D Lookup Table3/1 -> Gain3/1
  Gain2/1 -> Add/4
  1-D Lookup Table2/1 -> Gain2/1
  Gain1/1 -> Add/3
  1-D Lookup Table1/1 -> Gain1/1
  Gain6/1 -> Add/2
  1-D Lookup Table/1 -> Gain6/1
  Fcn/1 -> Add/1
  Clock/1 -> 1-D Lookup Table5/1, 1-D Lookup Table4/1, 1-D Lookup Table3/1, 1-D Lookup Table2/1, 1-D Lookup Table1/1, 1-D Lookup Table/1, Fcn/1
  connections:
  w/RConn1 -- PS-Simulink Converter1/LConn1 -- Hard_Stop_Ankle_L1/LConn1
  Hard_Stop_Ankle_L1/RConn1 -- PS Add/LConn2
  t/RConn1 -- PS Add1/RConn1
  q/RConn1 -- PS-Simulink Converter2/LConn1
  PS Add/RConn1 -- PS Add1/LConn1
  Simulink-PS Converter1/RConn1 -- PS Add1/LConn2
  Simulink-PS Converter2/RConn1 -- PS Add/LConn1

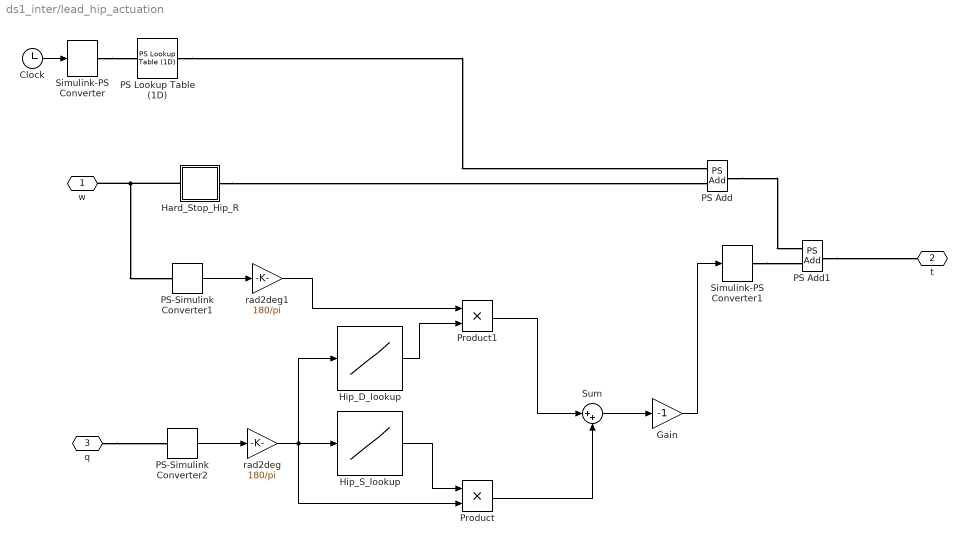
== system ds1_inter/lead_hip_actuation ==
  Clock : Clock
  Gain : Gain  Gain=-1
  Hard_Stop_Hip_R : Subsystem  mask{upper_bound=((125-p_swing_hip_i)*pi)/180, lower_bound=((-30-p_swing_hip_i)*pi)/180, contact_stiffness=1e8, contact_damping=5000, initial_angular_position=0}
      mask prompts: upper_bound "Upper Bound"; lower_bound "Lower Bound"; contact_stiffness "Contact Stiffness"; contact_damping "Contact Damping"; initial_angular_position "Initial Angular Position"
  Hip_D_lookup : Lookup_n-D  NumberOfTableDimensions=1  BreakpointsForDimension1=[-30:.01:125]  Table=[exp(linspace(log(1000),log(.01),1000)), zeros(1,13500),exp(linspace(log(.01),log(1000),1001))]  RndMeth=Simplest  InputSameDT=on
  Hip_S_lookup : Lookup_n-D  NumberOfTableDimensions=1  BreakpointsForDimension1=[-30:.01:125]  Table=[exp(linspace(log(10000),log(.01),1000)), zeros(1,13500),exp(linspace(log(.01),log(10000),1001))]  RndMeth=Simplest  InputSameDT=on
  PS Add : fl_ps_legacy_lib/Legacy Physical Signals/Functions/PS Add
      settings: SourceProductName=Simscape  SourceProductBaseCode=SS
  PS Add1 : fl_ps_legacy_lib/Legacy Physical Signals/Functions/PS Add
      settings: SourceProductName=Simscape  SourceProductBaseCode=SS
  PS Lookup Table (1D) : fl_ps_legacy_lib/Legacy Physical Signals/Lookup Tables/PS Lookup Table (1D)  x=linspace(0,.1667,21)'  f=(-M.strike_hip/1000)*bodymass  interp_method=2  extrap_method=1
      settings: SourceProductName=Simscape  SourceProductBaseCode=SS
  PS-Simulink Converter1 : nesl_utility/PS-Simulink Converter  PhysicalDomain=network_engine_domain  SubClassName=ps_output  LeftPortType=input  RightPortType=output  PseudoPeriodic=off  Frequencies=[]  Unit=1  AffineConversion=off
  PS-Simulink Converter2 : nesl_utility/PS-Simulink Converter  PhysicalDomain=network_engine_domain  SubClassName=ps_output  LeftPortType=input  RightPortType=output  PseudoPeriodic=off  Frequencies=[]  Unit=1  AffineConversion=off
  Product : Product  RndMeth=Zero
  Product1 : Product  RndMeth=Zero
  Simulink-PS Converter : nesl_utility/Simulink-PS Converter  PhysicalDomain=network_engine_domain  SubClassName=ps_input  LeftPortType=input  RightPortType=output  PseudoPeriodic=off  Frequencies=[]  NoiseDistribution=none  NoiseParameters=[]  Unit=1  AffineConversion=off  FilteringAndDerivatives=zero  SimscapeFilterOrder=1  InputFilterTimeConstant=.001  UdotUserProvided=[]
  Simulink-PS Converter1 : nesl_utility/Simulink-PS Converter  PhysicalDomain=network_engine_domain  SubClassName=ps_input  LeftPortType=input  RightPortType=output  PseudoPeriodic=off  Frequencies=[]  NoiseDistribution=none  NoiseParameters=[]  Unit=1  AffineConversion=off  FilteringAndDerivatives=zero  SimscapeFilterOrder=1  InputFilterTimeConstant=.001  UdotUserProvided=[]
  Sum : Sum  Inputs=|++
  rad2deg : Gain  Gain=180/pi
  "rad2deg1 " : Gain  Gain=180/pi
  w : PMIOPort  Side=Right
  t : PMIOPort  Port=2  Side=Left
  q : PMIOPort  Port=3  Side=Right
  wires:
  Clock/1 -> Simulink-PS Converter/1
  PS-Simulink Converter1/1 -> "rad2deg1 "/1
  PS-Simulink Converter2/1 -> rad2deg/1
  rad2deg/1 -> Hip_S_lookup/1, Hip_D_lookup/1, Product/2
  Hip_S_lookup/1 -> Product/1
  "rad2deg1 "/1 -> Product1/1
  Product1/1 -> Sum/1
  Product/1 -> Sum/2
  Sum/1 -> Gain/1
  Gain/1 -> Simulink-PS Converter1/1
  Hip_D_lookup/1 -> Product1/2
  connections:
  Hard_Stop_Hip_R/RConn1 -- PS Add/LConn2
  Hard_Stop_Hip_R/LConn1 -- PS-Simulink Converter1/LConn1 -- w/RConn1
  Simulink-PS Converter/RConn1 -- PS Lookup Table (1D)/LConn1
  q/RConn1 -- PS-Simulink Converter2/LConn1
  PS Add/RConn1 -- PS Add1/LConn1
  PS Add1/RConn1 -- t/RConn1
  PS Lookup Table (1D)/RConn1 -- PS Add/LConn1
  Simulink-PS Converter1/RConn1 -- PS Add1/LConn2
